simulink model "hydraulic"  (R2025b)
settings: Solver=FixedStepAuto  StartTime=0.0  StopTime=5  RelTol=1e-3
model workspace (MAT data in the model file):
  Ap = 0.0314
  Ct = 2.4e-12
  Fforce = 90000
  Gmass = 9000
  Kc = 1.68e-09
  Kq = 1.63
  L_init = 0.1
  Ve = 0.11304
  beta_e = 700000000
settings Model: ParameterArgumentNames=Ap,Ct,Fforce,Gmass,Kc,Kq,L_init,Ve,beta_e  Creator=LYG  LastModifiedBy=LYG

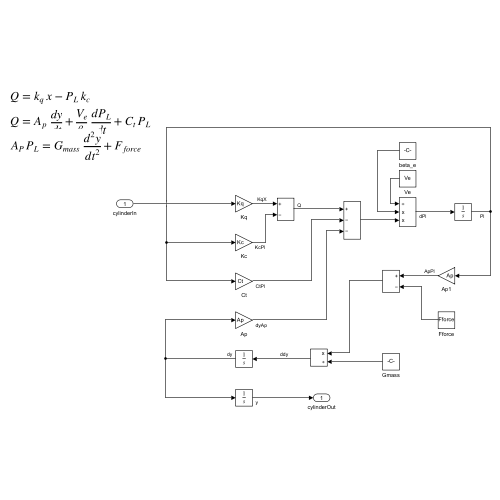
[thumbnail: Simulink's stored preview of the top-level diagram]
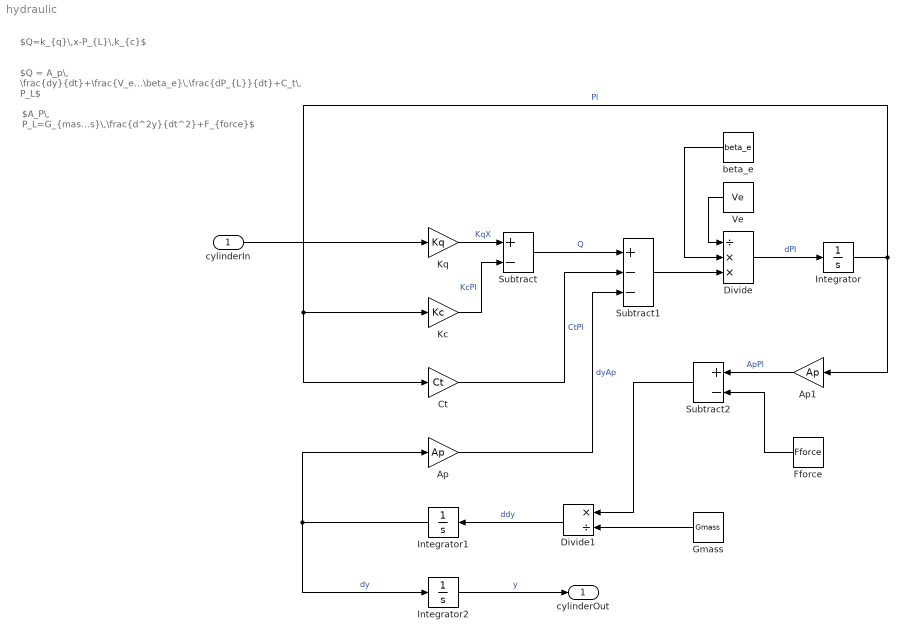
== system hydraulic ==
  note: $A_P\, P_L=G_{mass}\,\frac{d^2y}{dt^2}+F_{force}$
  note: $Q = A_p\, \frac{dy}{dt}+\frac{V_e}{\beta_e}\,\frac{dP_{L}}{dt}+C_t\, P_L$
  note: $Q=k_{q}\,x-P_{L}\,k_{c}$
  cylinderIn : Inport
  Ap : Gain  Gain=Ap
  Ap1 : Gain  Gain=Ap
  Ct : Gain  Gain=Ct
  Divide : Product  Inputs=/**
  Divide1 : Product  Inputs=*/
  Fforce : Constant  Value=Fforce
  Gmass : Constant  Value=Gmass
  Integrator : Integrator  InitialCondition=Fforce / Ap
  Integrator1 : Integrator
  Integrator2 : Integrator  InitialCondition=L_init
  Kc : Gain  Gain=Kc
  Kq : Gain  Gain=Kq
  Subtract : Sum  Inputs=+-
  Subtract1 : Sum  Inputs=+--
  Subtract2 : Sum  Inputs=+-
  Ve : Constant  Value=Ve
  beta_e : Constant  Value=beta_e
  cylinderOut : Outport
  wires:
  Kq/1 -> Subtract/1  "KqX"
  Subtract/1 -> Subtract1/1  "Q"
  Ap/1 -> Subtract1/3  "dyAp"
  Integrator1/1 -> Integrator2/1, Ap/1  "dy"
  Integrator/1 -> Ct/1, Kc/1, Ap1/1  "Pl"
  Kc/1 -> Subtract/2  "KcPl"
  Ct/1 -> Subtract1/2  "CtPl"
  Subtract1/1 -> Divide/3
  beta_e/1 -> Divide/2
  Ve/1 -> Divide/1
  Divide/1 -> Integrator/1  "dPl"
  Divide1/1 -> Integrator1/1  "ddy"
  Ap1/1 -> Subtract2/1  "ApPl"
  Fforce/1 -> Subtract2/2
  Subtract2/1 -> Divide1/1
  Gmass/1 -> Divide1/2
  Integrator2/1 -> cylinderOut/1  "y"
  cylinderIn/1 -> Kq/1
